simulink model "Atomic_Subsystem0"  (R2020b)
settings: Solver=VariableStepAuto  StartTime=0.0  StopTime=120  RelTol=1e-3
model workspace (MAT data in the model file):
  b = 50
  m = 1000
settings Model: DataDictionary=parameter3.sldd  Creator=Puru Gawande  LastModifiedBy=Puru Gawande
settings DataIOCC: SaveOutput=off  SaveTime=off

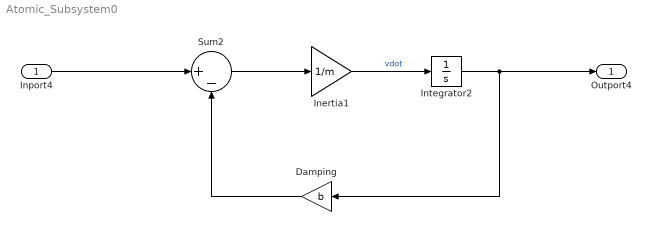
== system Atomic_Subsystem0 ==
  Inport4 : Inport
  Damping : Gain  Gain=b
  Inertia1 : Gain  Gain=1/m
  Integrator2 : Integrator
  Sum2 : Sum  Inputs=|+-
  Outport4 : Outport
  wires:
  Integrator2/1 -> Outport4/1, Damping/1
  Inport4/1 -> Sum2/1
  Sum2/1 -> Inertia1/1
  Inertia1/1 -> Integrator2/1  "vdot"
  Damping/1 -> Sum2/2
